simulink model "Discrete_Time_falling_verif"  (Simulink 8.4)
settings: Solver=ode45  StartTime=0.0  StopTime=10.0  RelTol=1e-3
undefined symbols (not defined in the file): DiscIntNeverNeededParam, sigbuilder_block
settings Model: Creator=Romain  LastModifiedBy=hbourbou
settings DataIOCC: SignalLoggingSaveFormat=Dataset
settings OptimizationCC: ExpressionDepthLimit=128
settings DebuggingCC: SolverPrmCheckMsg=none  FcnCallInpInsideContextMsg=EnableAllAsError  FrameProcessingCompatibilityMsg=error  StateNameClashWarn=none
settings GRTTargetCC: CombineOutputUpdateFcns=on  GRTInterface=off

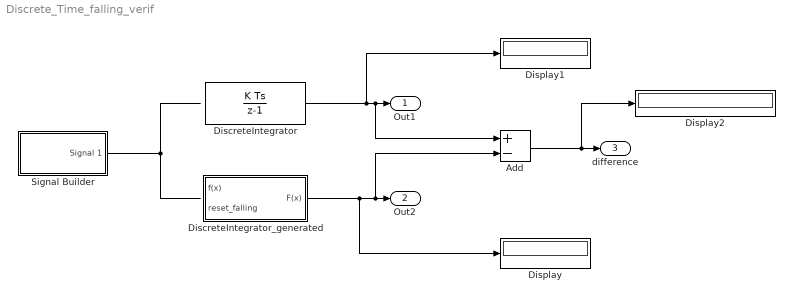
== system Discrete_Time_falling_verif ==
  Add : Sum  Inputs=+-
  DiscreteIntegrator : DiscreteIntegrator  ExternalReset=falling  InitialConditionSetting=State (most efficient)  SampleTime=-1  ICPrevOutput=DiscIntNeverNeededParam  ICPrevScaledInput=DiscIntNeverNeededParam
  DiscreteIntegrator_generated : Subsystem  TreatAsAtomicUnit=on
  Display : Display
  Display1 : Display
  Display2 : Display
  Signal Builder : Subsystem  Tag=STV Subsys  LoadFcn=sigbuilder_block('load');  StartFcn=sigbuilder_block('start');  StopFcn=sigbuilder_block('stop');  ClipboardFcn=sigbuilder_block('clipboard');  mask(Sigbuilder block){}
      mask help: Simulink:masks:SigbuilderBlock_MD
      mask init:
      | if ~strcmp(get_param(bdroot(gcbh),'SimulationStatus'),'stopped') tuvar = sigbuilder_block('maskInit'); end
      settings: CopyFcn=sigbuilder_block('copy');  DeleteFcn=sigbuilder_block('delete');  ModelCloseFcn=sigbuilder_block('modelClose');  PreSaveFcn=sigbuilder_block('preSave');  PauseFcn=sigbuilder_block('pause');  ContinueFcn=sigbuilder_block('continue');  NameChangeFcn=sigbuilder_block('namechange');  OpenFcn=sigbuilder_block('open',[437.6 199.2 550.4 400 ]);  CloseFcn=sigbuilder_block('close');
      mask Display: plot(0, 0, 100, 100,[2, 2, 32, 32, 2], [68, 8, 8, 68, 68],[32, 2], [38, 38], [32, 19, 2],[53, 60, 44], [32, 17, 17, 2],[16, 16, 31, 31]);txt = getActiveGroup(gcbh);text(2, 100, txt,'verticalAlignment', 'top');
  Out1 : Outport
  Out2 : Outport  Port=2
  difference : Outport  Port=3
  wires:
  Signal Builder/1(Signal 1) -> ?
  DiscreteIntegrator/1 -> Display1/1, Add/1, Out1/1
  DiscreteIntegrator_generated/1(F(x)) -> Display/1, Add/2, Out2/1
  Add/1 -> Display2/1, difference/1

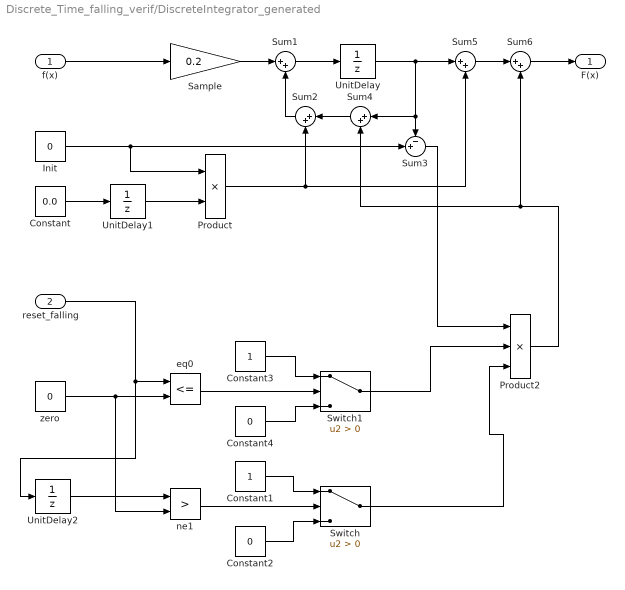
== system Discrete_Time_falling_verif/DiscreteIntegrator_generated ==
  f(x) : Inport
  reset_falling : Inport  Port=2
  Constant : Constant  Value=0.0  SampleTime=-1
  Constant1 : Constant
  Constant2 : Constant  Value=0
  Constant3 : Constant
  Constant4 : Constant  Value=0
  Init : Constant  Value=0  SampleTime=-1
  Product : Product  RndMeth=Zero
  Product2 : Product  Inputs=3  RndMeth=Zero
  Sample : Gain  Gain=0.2
  Sum1 : Sum  RequirementInfo={} %GIDa_0a25cdb1_03db_423e_a71f_300b95199d3f  Inputs=|++
  Sum2 : Sum  RequirementInfo={} %GIDa_95d01b60_89a6_4238_922c_ec8ca4bf52e2  Inputs=|++
  Sum3 : Sum  RequirementInfo={} %GIDa_47f5dd6c_39ea_4bda_860f_2292fe6f5ac1  Inputs=-+|
  Sum4 : Sum  RequirementInfo={} %GIDa_b07dfc36_01d3_41c6_8f25_ede4b66b530e  Inputs=|++
  Sum5 : Sum  RequirementInfo={} %GIDa_ba422a1e_7fea_4ab6_8be4_d1e4e8af7d0d  Inputs=|++
  Sum6 : Sum  RequirementInfo={} %GIDa_be8d8ac6_df1c_457d_a9cd_7ec9464535e5  Inputs=|++  SampleTime=0.2
  Switch : Switch  Criteria=u2 > Threshold
  Switch1 : Switch  Criteria=u2 > Threshold
  UnitDelay : UnitDelay  SampleTime=0.2
  UnitDelay1 : UnitDelay  InitialCondition=1  SampleTime=0.2
  UnitDelay2 : UnitDelay  SampleTime=0.2
  eq0 : RelationalOperator  Operator=<=  OutDataTypeStr=boolean
  ne1 : RelationalOperator  Operator=>  OutDataTypeStr=boolean
  zero : Constant  Value=0  SampleTime=-1
  F(x) : Outport  RequirementInfo={} %GIDa_c1120e5e_cddf_421c_9520_2f690319ee41
  wires:
  Sum1/1 -> UnitDelay/1
  Sample/1 -> Sum1/1
  UnitDelay/1 -> Sum5/1, Sum3/1, Sum4/1
  Sum2/1 -> Sum1/2
  Product/1 -> Sum5/2, Sum2/2
  UnitDelay1/1 -> Product/2
  Constant/1 -> UnitDelay1/1
  Init/1 -> Product/1, Sum3/2
  reset_falling/1 -> UnitDelay2/1, eq0/1
  UnitDelay2/1 -> ne1/1
  Sum3/1 -> Product2/1
  zero/1 -> ne1/2, eq0/2
  Sum4/1 -> Sum2/1
  Product2/1 -> Sum6/2, Sum4/2
  f(x)/1 -> Sample/1
  Sum5/1 -> Sum6/1
  Sum6/1 -> F(x)/1
  ne1/1 -> Switch/2
  Constant1/1 -> Switch/1
  Constant2/1 -> Switch/3
  Switch/1 -> Product2/3
  eq0/1 -> Switch1/2
  Constant3/1 -> Switch1/1
  Constant4/1 -> Switch1/3
  Switch1/1 -> Product2/2

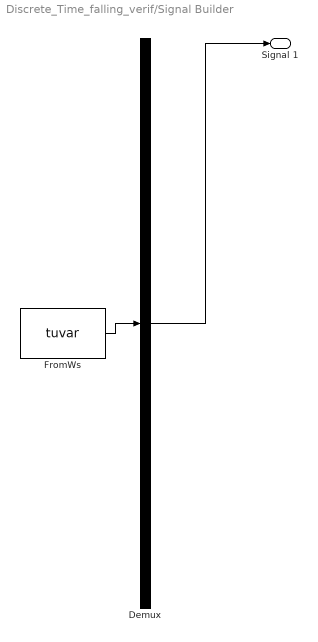
== system Discrete_Time_falling_verif/Signal Builder ==
  Demux : Demux  Tag=STV Demux  Outputs=1
  FromWs : FromWorkspace  Tag=STV FromWs  VariableName=tuvar  SampleTime=0  SigBuilderData=DataTag0  VnvData=DataTag1
      SigBuilderData=|
      | common.afterFinalStr = 'Extrapolate'
      | common.sampleTime = 0
      | dataSet.timeRange = [0 10]
      | dataSet.name = 'Group 1'
      | sbobj.Groups.Name = 'Group 1'
      | sbobj.Groups.Signals.Name = 'Signal 1'
      | sbobj.Groups.Signals.XData = [0 4 4 6 6 10]
      | sbobj.Groups.Signals.YData = [0 0.99 1 0.3 0.26 0]
  Signal 1 : Outport  Tag=STV Outport
  wires:
  Demux/1 -> Signal 1/1
  FromWs/1 -> Demux/1
